simulink model "Sim_Multi"  (R2016b)
settings: Solver=ode3  StartTime=0.0  StopTime=sim_time  FixedStep=t_sim  MaxStep=t_control  RelTol=1e-5  EnableMultiTasking=on
values from neighbouring files (symbols this model uses):
  Att_init = [0;0;0] * d2r    [Init_Multi.m]
  Blade_flapping = 0    [Init_Multi.m]
  C_D = 0.40    (= 0.4)    [Init_Multi.m]
  CoG_nominal = [0;0;0.001]    [Init_Multi.m]
  CoG_real = [0;0;0.001]    [Init_Multi.m]
  Coriolis_correction = 1    [Init_Multi.m]
  d2r = pi/180    (= 0.0174532925199)    [Init_Multi.m]
  Dyn_thrust = 0    [Init_Multi.m]
  g = 9.80665    [Init_Multi.m]
  J_nominal = [Jxx Jxy Jxz;Jyx Jyy Jyz;Jzx Jzy Jzz]    [Init_Multi.m]
  J_real = [Jxx Jxy Jxz;Jyx Jyy Jyz;Jzx Jzy Jzz]    [Init_Multi.m]
  k1 = -1.125    [Init_Multi.m]
  k2 = -1.372    [Init_Multi.m]
  k3 = -1.718    [Init_Multi.m]
  k4 = -0.655    [Init_Multi.m]
  k_a1s = 1.5 / 4.0    (= 0.375)    [Init_Multi.m]
  k_beta = 0.23    [Init_Multi.m]
  kappa = 1.00    (= 1)    [Init_Multi.m]
  Kff_1 = 0.7*[1;1;0.95]    [Init_Multi.m]
  Ki_1 = 10*[1;1;1.5]    [Init_Multi.m]
  Kp_1 = 15*[1;1;1.5]    [Init_Multi.m]
  mass_nominal = 0.550    (= 0.55)    [Init_Multi.m]
  mass_real = 0.550    (= 0.55)    [Init_Multi.m]
  max_thrust = max_thrust + (MotorMatrix_nominal(i,7)*MotorMatrix_nominal(i,12)+MotorMatrix_nominal(i,8)*MotorMatrix_nominal(i,12)^2)    [Init_Multi.m]
  MaxRate_cmd = [360;360;120] * d2r    [Init_Multi.m]
  min_thrust = min_thrust + (MotorMatrix_nominal(i,7)*MotorMatrix_nominal(i,11)+MotorMatrix_nominal(i,8)*MotorMatrix_nominal(i,11)^2)    [Init_Multi.m]
  MotorMap = B' * inv(B * B')    [Init_Multi.m]
  MotorMatrix_nominal = [045 , 0.170 , -0.028 , -1 , 1.0 , 0.010 , [9.6820 , 0.010872]*1e-5 , [1.4504 , 0.0016312]*1e-6 , 0000 , 6000 , [0.0 , 0.0 , 0.0] , 8*2.54/100 , 11/1000;                         135 , 0.170 , -0.028 , +1 , 1.0 , 0.010 , [9.6820 , 0.010872]*1e-5 , [1.4504 , 0.0016312]*1e-6 , 0000 , 6000 , [0.0 , 0.0 , 0.0] , 8*2.54/100 , 11/1000;                         225 , 0.170 , -0.028 , -1 , 1.0 , 0.010 , [9. ...(+284 chars)    [Init_Multi.m]
  MotorMatrix_real = [045 , 0.170 , -0.028 , -1 , 1.0 , 0.010 , [9.6820 , 0.010872]*1e-5 , [1.4504 , 0.0016312]*1e-6 , 0000 , 6000 , [0.0 , 0.0 , 0.0] , 8*2.54/100 , 11/1000;                      135 , 0.170 , -0.028 , +1 , 1.0 , 0.010 , [9.6820 , 0.010872]*1e-5 , [1.4504 , 0.0016312]*1e-6 , 0000 , 6000 , [0.0 , 0.0 , 0.0] , 8*2.54/100 , 11/1000;                      225 , 0.170 , -0.028 , -1 , 1.0 , 0.010 , [9.6820 , ...(+275 chars)    [Init_Multi.m]
  Noise_flag = 0    [Init_Multi.m]
  omega_init = [0;0;0]    [Init_Multi.m]
  q_init = rpy2quat(Att_init)    [Init_Multi.m]
  r2d = 180/pi    (= 57.2957795131)    [Init_Multi.m]
  rho = 1.225    [Init_Multi.m]
  rpm2radpersec = 2*pi/60    (= 0.10471975512)    [Init_Multi.m]
  rpm_init = 3104.5025852    [Init_Multi.m]
  Surface_params = [a;b;c]    [Init_Multi.m]
  t_control = 1/500    (= 0.002)    [Init_Multi.m]
  t_sim = t_control/2    (= 0.001)    [Init_Multi.m]
  thrust_gain = (max_thrust - min_thrust) / 1000    (= 0)    [Init_Multi.m]
  thrust_offset = min_thrust    (= 0)    [Init_Multi.m]
  thrust_reserve = 0.10    (= 0.1)    [Init_Multi.m]
  v_h = 4.0    (= 4)    [Init_Multi.m]
  Vb_init = [0;0;0]    [Init_Multi.m]
  Vi_init = R_IB_init' * Vb_init    [Init_Multi.m]
  Xi_init = [0;0;0]    [Init_Multi.m]
undefined symbols (not defined in the file or in its folder): DiscIntNeverNeededParam, rpy2quat, thrust2rpm
libraries: simulink x17
(part 3 of 4)

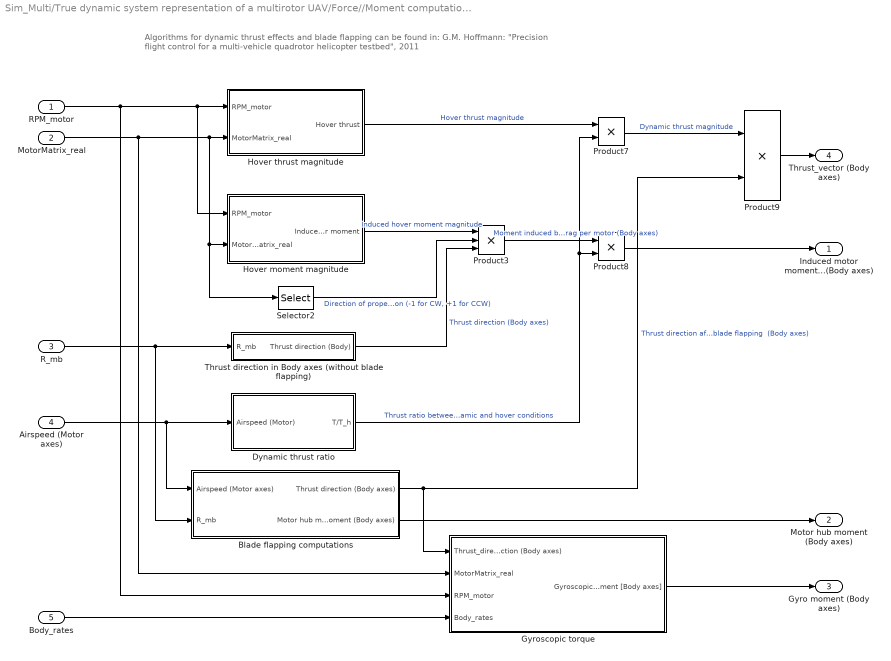
== system Sim_Multi/True dynamic system representation of a multirotor UAV/Force//Moment computation/Forces and moments generated by spinning propellers/For Each Subsystem/Thrust//moment vector for each propeller (Body axes)/Compute dynamic motor thrust and moments ==
  note: Algorithms for dynamic thrust effects and blade flapping can be found in:
      | G.M. Hoffmann: "Precision flight control for a multi-vehicle quadrotor helicopter testbed", 2011
  RPM_motor : Inport
  MotorMatrix_real : Inport  Port=2
  R_mb : Inport  Port=3
  Airspeed (Motor axes) : Inport  Port=4
  Body_rates : Inport  Port=5
  Blade flapping computations : Subsystem
  Dynamic thrust ratio : Subsystem
  Gyroscopic torque : Subsystem
  Hover moment magnitude : Subsystem
  Hover thrust magnitude : Subsystem
  Product3 : Product  Inputs=3
  Product7 : Product
  Product8 : Product
  Product9 : Product
  Selector2 : Selector  InputPortWidth=17  IndexOptions=Index vector (dialog)  Indices=[4]  OutputSizes=1
  Thrust direction in Body axes (without blade flapping) : Subsystem
  Induced motor moment (Body axes) : Outport
  Motor hub moment (Body axes) : Outport  Port=2
  Gyro moment (Body axes) : Outport  Port=3
  Thrust_vector (Body axes) : Outport  Port=4
  wires:
  RPM_motor/1 -> Gyroscopic torque/3(RPM_motor), Hover moment magnitude/1(RPM_motor), Hover thrust magnitude/1(RPM_motor)
  MotorMatrix_real/1 -> Gyroscopic torque/2(MotorMatrix_real), Selector2/1, Hover moment magnitude/2(MotorMatrix_real), Hover thrust magnitude/2(MotorMatrix_real)
  Selector2/1 -> Product3/2  "Direction of propeller rotation (-1 for CW, +1 for CCW)"
  Thrust direction in Body axes (without blade flapping)/1(Thrust direction (Body)) -> Product3/3  "Thrust direction (Body axes)"
  R_mb/1 -> Blade flapping computations/2(R_mb), Thrust direction in Body axes (without blade flapping)/1(R_mb)
  Airspeed (Motor axes)/1 -> Blade flapping computations/1(Airspeed (Motor axes)), Dynamic thrust ratio/1(Airspeed (Motor))
  Product3/1 -> Product8/1  "Moment induced by aerodynamic drag per motor (Body axes)"
  Product8/1 -> Induced motor moment (Body axes)/1
  Product7/1 -> Product9/1  "Dynamic thrust magnitude"
  Product9/1 -> Thrust_vector (Body axes)/1
  Blade flapping computations/1(Thrust direction (Body axes)) -> Gyroscopic torque/1(Thrust_direction (Body axes)), Product9/2  "Thrust direction after blade flapping  (Body axes)"
  Blade flapping computations/2(Motor hub moment (Body axes)) -> Motor hub moment (Body axes)/1
  Body_rates/1 -> Gyroscopic torque/4(Body_rates)
  Gyroscopic torque/1(Gyroscopic moment [Body axes]) -> Gyro moment (Body axes)/1
  Hover thrust magnitude/1(Hover thrust) -> Product7/1  "Hover thrust magnitude"
  Hover moment magnitude/1(Induced hover moment) -> Product3/1  "Induced hover moment magnitude"
  Dynamic thrust ratio/1(T/T_h) -> Product7/2, Product8/2  "Thrust ratio between dynamic and hover conditions"

== system Sim_Multi/True dynamic system representation of a multirotor UAV/Force//Moment computation/Forces and moments generated by spinning propellers/For Each Subsystem/Thrust//moment vector for each propeller (Body axes)/Coordinate transformation Body to Motor axes ==
  note: The true airspeed at prop computed here is the linear velocity (now in Motor axes)
      | with which this particular motor moves through the air.
      | So the point of view is: the surrounding air standing still and the airframe moving through it.
  MotorMatrix_real : Inport
  Airspeed (Body axes) : Inport  Port=2
  Conversion deg to rad : Gain  Gain=d2r
  Product : Product  Multiplication=Matrix(*)
  Rotation Matrix Body to Motor : Subsystem
  Selector : Selector  InputPortWidth=17  IndexOptions=Index vector (dialog)  Indices=[13 14 15]  OutputSizes=1
  R_mb : Outport
  Airspeed (Motor axes) : Outport  Port=2
  wires:
  Product/1 -> Airspeed (Motor axes)/1  "True airspeed at prop (Motor axes)"
  Rotation Matrix Body to Motor/1(R_mb) -> R_mb/1, Product/1  "Rotation matrix Body to Motor axes"
  MotorMatrix_real/1 -> Selector/1
  Selector/1 -> Conversion deg to rad/1
  Airspeed (Body axes)/1 -> Product/2  "True airspeed at prop (Body axes)"
  Conversion deg to rad/1 -> Rotation Matrix Body to Motor/1(Motor angles)

== system Sim_Multi/True dynamic system representation of a multirotor UAV/Force//Moment computation/Forces and moments generated by spinning propellers/For Each Subsystem/Thrust//moment vector for each propeller (Body axes)/Cross Product ==
  u : Inport
  v : Inport  Port=2
  Subsystem : Subsystem
  Subsystem1 : Subsystem
  Sum : Sum  Inputs=+|-
  u x v : Outport
  wires:
  Sum/1 -> u x v/1
  u/1 -> Subsystem1/1(u), Subsystem/1(u)
  v/1 -> Subsystem1/2(v), Subsystem/2(v)
  Subsystem/1(Positive elements) -> Sum/1
  Subsystem1/1(Negative elements) -> Sum/2

== system Sim_Multi/Controller/Controller Structure/Inner-loop control only/PI Rate controller/Gain Kff/Create diagonal 3x3 matrix/Subsystem9 ==
  C_11 : Inport  PortDimensions=1
  C_12 : Inport  Port=2  PortDimensions=1
  C_13 : Inport  Port=3  PortDimensions=1
  C_21 : Inport  Port=4  PortDimensions=1
  C_22 : Inport  Port=5  PortDimensions=1
  C_23 : Inport  Port=6  PortDimensions=1
  C_31 : Inport  Port=7  PortDimensions=1
  C_32 : Inport  Port=8  PortDimensions=1
  C_33 : Inport  Port=9  PortDimensions=1
  Reshape (9) to [3x3] column-major : Reshape  OutputDimensionality=Customize  OutputDimensions=[3,3]
  Vector Concatenate : Concatenate  NumInputs=9
  Diag : Outport
  wires:
  C_33/1 -> Vector Concatenate/9
  C_22/1 -> Vector Concatenate/5
  Reshape (9) to [3x3] column-major/1 -> Diag/1
  C_11/1 -> Vector Concatenate/1
  Vector Concatenate/1 -> Reshape (9) to [3x3] column-major/1
  C_32/1 -> Vector Concatenate/6
  C_31/1 -> Vector Concatenate/3
  C_21/1 -> Vector Concatenate/2
  C_13/1 -> Vector Concatenate/7
  C_12/1 -> Vector Concatenate/4
  C_23/1 -> Vector Concatenate/8

== system Sim_Multi/Controller/Controller Structure/Inner-loop control only/PI Rate controller/Gain Ki/Create diagonal 3x3 matrix/Subsystem9 ==
  C_11 : Inport  PortDimensions=1
  C_12 : Inport  Port=2  PortDimensions=1
  C_13 : Inport  Port=3  PortDimensions=1
  C_21 : Inport  Port=4  PortDimensions=1
  C_22 : Inport  Port=5  PortDimensions=1
  C_23 : Inport  Port=6  PortDimensions=1
  C_31 : Inport  Port=7  PortDimensions=1
  C_32 : Inport  Port=8  PortDimensions=1
  C_33 : Inport  Port=9  PortDimensions=1
  Reshape (9) to [3x3] column-major : Reshape  OutputDimensionality=Customize  OutputDimensions=[3,3]
  Vector Concatenate : Concatenate  NumInputs=9
  Diag : Outport
  wires:
  C_33/1 -> Vector Concatenate/9
  C_22/1 -> Vector Concatenate/5
  Reshape (9) to [3x3] column-major/1 -> Diag/1
  C_11/1 -> Vector Concatenate/1
  Vector Concatenate/1 -> Reshape (9) to [3x3] column-major/1
  C_32/1 -> Vector Concatenate/6
  C_31/1 -> Vector Concatenate/3
  C_21/1 -> Vector Concatenate/2
  C_13/1 -> Vector Concatenate/7
  C_12/1 -> Vector Concatenate/4
  C_23/1 -> Vector Concatenate/8

== system Sim_Multi/Controller/Controller Structure/Inner-loop control only/PI Rate controller/Gain Kp/Create diagonal 3x3 matrix/Subsystem9 ==
  C_11 : Inport  PortDimensions=1
  C_12 : Inport  Port=2  PortDimensions=1
  C_13 : Inport  Port=3  PortDimensions=1
  C_21 : Inport  Port=4  PortDimensions=1
  C_22 : Inport  Port=5  PortDimensions=1
  C_23 : Inport  Port=6  PortDimensions=1
  C_31 : Inport  Port=7  PortDimensions=1
  C_32 : Inport  Port=8  PortDimensions=1
  C_33 : Inport  Port=9  PortDimensions=1
  Reshape (9) to [3x3] column-major : Reshape  OutputDimensionality=Customize  OutputDimensions=[3,3]
  Vector Concatenate : Concatenate  NumInputs=9
  Diag : Outport
  wires:
  C_33/1 -> Vector Concatenate/9
  C_22/1 -> Vector Concatenate/5
  Reshape (9) to [3x3] column-major/1 -> Diag/1
  C_11/1 -> Vector Concatenate/1
  Vector Concatenate/1 -> Reshape (9) to [3x3] column-major/1
  C_32/1 -> Vector Concatenate/6
  C_31/1 -> Vector Concatenate/3
  C_21/1 -> Vector Concatenate/2
  C_13/1 -> Vector Concatenate/7
  C_12/1 -> Vector Concatenate/4
  C_23/1 -> Vector Concatenate/8

== system Sim_Multi/True dynamic system representation of a multirotor UAV/Force//Moment computation/Compute aerodynamic drag of the airframe in Body axes/Aerodynamic drag force/Nonzero airspeed/Normalize/norm ==
  u : Inport
  Complex to Real-Imag : ComplexToRealImag  Output=Real
  Sqrt : Sqrt  SaturateOnIntegerOverflow=on
  dot_product : Subsystem
  ||u|| : Outport
  wires:
  u/1 -> dot_product/1(u), dot_product/2(v)
  dot_product/1(u.v) -> Sqrt/1
  Sqrt/1 -> Complex to Real-Imag/1
  Complex to Real-Imag/1 -> ||u||/1

== system Sim_Multi/True dynamic system representation of a multirotor UAV/Force//Moment computation/Compute aerodynamic drag of the airframe in Body axes/Aerodynamic drag force/Nonzero airspeed/Surface area computation/Scaling factor computation ==
  Airspeed (Body) : Inport
  Surface_params : Inport  Port=2
  Add : Sum  Inputs=+++
  Demux : Demux  Outputs=3
  Demux1 : Demux  Outputs=3
  Divide : Product  Inputs=*/
  Divide1 : Product  Inputs=*/
  Divide2 : Product  Inputs=*/
  Product : Product
  Product1 : Product
  Product2 : Product
  Reciprocal Sqrt : Sqrt  Operator=rSqrt  SaturateOnIntegerOverflow=on
  Scaling factor : Outport
  wires:
  Divide2/1 -> Product2/2, Product2/1
  Reciprocal Sqrt/1 -> Scaling factor/1
  Demux1/3 -> Divide2/2  "c"
  Demux/3 -> Divide2/1  "z"
  Divide/1 -> Product/2, Product/1
  Airspeed (Body)/1 -> Demux/1
  Surface_params/1 -> Demux1/1
  Demux1/1 -> Divide/2  "a"
  Demux/1 -> Divide/1  "x"
  Product/1 -> Add/1
  Product2/1 -> Add/3
  Add/1 -> Reciprocal Sqrt/1
  Demux/2 -> Divide1/1  "y"
  Divide1/1 -> Product1/2, Product1/1
  Demux1/2 -> Divide1/2  "b"
  Product1/1 -> Add/2

== system Sim_Multi/True dynamic system representation of a multirotor UAV/Force//Moment computation/Compute aerodynamic drag of the airframe in Body axes/Aerodynamic drag force/Nonzero airspeed/Surface area computation/Surface area computation ==
  Airspeed (Body) : Inport
  Scaling factor : Inport  Port=2
  Product : Product
  norm : Subsystem
  Surface area : Outport
  wires:
  Scaling factor/1 -> Product/2
  Airspeed (Body)/1 -> Product/1
  Product/1 -> norm/1(u)
  norm/1(||u||) -> Surface area/1

== system Sim_Multi/True dynamic system representation of a multirotor UAV/Force//Moment computation/Compute aerodynamic drag of the airframe in Body axes/Aerodynamic drag force/Nonzero airspeed/u^2/dot_product ==
  u : Inport
  v : Inport  Port=2
  Product : Product  Multiplication=Matrix(*)  RndMeth=Zero
  Reshape : Reshape  OutputDimensionality=Column vector (2-D)
  Reshape1 : Reshape  OutputDimensionality=Column vector (2-D)
  transpose : Math  Operator=transpose  SaturateOnIntegerOverflow=on
  u.v : Outport
  wires:
  v/1 -> Reshape1/1
  u/1 -> Reshape/1
  Reshape/1 -> transpose/1
  transpose/1 -> Product/1
  Reshape1/1 -> Product/2
  Product/1 -> u.v/1

== system Sim_Multi/True dynamic system representation of a multirotor UAV/Force//Moment computation/Forces and moments generated by spinning propellers/For Each Subsystem/Thrust//moment vector for each propeller (Body axes)/Compute dynamic motor thrust and moments/Blade flapping computations ==
  note: Blade flapping computations are motivated by algorithms found in:
      | G.M. Hoffmann: "Precision flight control for a multi-vehicle quadrotor helicopter testbed", 2011
      | The idea is the following:
      | The thrust vector is tilted backwards from the direction of motion. The amount of tilt depends on the magnitude of the airspeed vector in the (untilted) propeller plane.
      | The tilt direction is in the plane defined by the airspeed xy vector and the (untilted) thrust vector in Motor axes.
      | The normal vector to this plane can be found by computing the cross product of untilted thrust vector and airspeed xy vector.
      | The new (tilted) thrust vector can then be found by applying the Rodrigues rotation formula, see Wikipedia
  Airspeed (Motor axes) : Inport
  R_mb : Inport  Port=2
  Demux4 : Demux  Outputs=[2,1]
  If : If  IfExpression=u1 == 0
  Merge : Merge
  Merge1 : Merge
  Nonzero airspeed in rotor plane : Subsystem  TreatAsAtomicUnit=on
  Terminator : Terminator
  Zero airspeed in rotor plane : Subsystem  TreatAsAtomicUnit=on
  norm : Subsystem
  Thrust direction (Body axes) : Outport
  Motor hub moment (Body axes) : Outport  Port=2
  wires:
  If/1 -> Zero airspeed in rotor plane/Action
  Zero airspeed in rotor plane/1(Thrust direction (Body)) -> Merge/1
  Nonzero airspeed in rotor plane/1(Thrust direction (Body)) -> Merge/2
  If/2 -> Nonzero airspeed in rotor plane/Action
  Airspeed (Motor axes)/1 -> Demux4/1
  Demux4/2 -> Terminator/1  "Airspeed component along motor shaft"
  Demux4/1 -> norm/1(u), Zero airspeed in rotor plane/1(Airspeed xy), Nonzero airspeed in rotor plane/1(Airspeed xy)  "Airspeed components in (unbent) rotor plane"
  norm/1(||u||) -> If/1  "Airspeed xy component  magnitude"
  Merge/1 -> Thrust direction (Body axes)/1  "New tilted thrust direction (Body axes) (This is a unit vector)"
  R_mb/1 -> Nonzero airspeed in rotor plane/2(R_mb), Zero airspeed in rotor plane/2(R_mb)
  Merge1/1 -> Motor hub moment (Body axes)/1  "Moment in the motor hub due to bending of the propeller (Body axes)"
  Zero airspeed in rotor plane/2(Hub moment (Body)) -> Merge1/1
  Nonzero airspeed in rotor plane/2(Hub moment (Body)) -> Merge1/2

== system Sim_Multi/True dynamic system representation of a multirotor UAV/Force//Moment computation/Forces and moments generated by spinning propellers/For Each Subsystem/Thrust//moment vector for each propeller (Body axes)/Compute dynamic motor thrust and moments/Dynamic thrust ratio ==
  Airspeed (Motor) : Inport
  Angle of attack and airspeed magnitude : Subsystem
  Compute the climb speed : Subsystem
  Constant : Constant
  Constant1 : Constant  Value=Dyn_thrust
  Divide : Product  Inputs=*/
  Flight modes of the propeller : Subsystem
  Induced velocity at hover : Constant  Value=v_h
  Product2 : Product
  Sum2 : Sum  Inputs=|+-
  Switch : Switch  Criteria=u2 > Threshold  Threshold=0.5
  Trigonometric Function : Trigonometry
  T/T_h : Outport
  wires:
  Airspeed (Motor)/1 -> Angle of attack and airspeed magnitude/1(Airspeed (Motor axes)), Compute the climb speed/1(Airspeed (Motor axes))
  Trigonometric Function/1 -> Product2/1
  Sum2/1 -> Divide/2
  Angle of attack and airspeed magnitude/2(Airspeed magnitude) -> Product2/2  "Airspeed magnitude v_inf"
  Angle of attack and airspeed magnitude/1(AoA (rad)) -> Trigonometric Function/1  "Angle of Attack"
  Compute the climb speed/1(v_c) -> Flight modes of the propeller/2(v_c)
  Flight modes of the propeller/1(v_i) -> Sum2/1
  Product2/1 -> Sum2/2
  Induced velocity at hover/1 -> Divide/1, Flight modes of the propeller/1(v_h)
  Switch/1 -> T/T_h/1  "Thrust ratio T/T_h"
  Divide/1 -> Switch/1
  Constant/1 -> Switch/3
  Constant1/1 -> Switch/2

== system Sim_Multi/True dynamic system representation of a multirotor UAV/Force//Moment computation/Forces and moments generated by spinning propellers/For Each Subsystem/Thrust//moment vector for each propeller (Body axes)/Compute dynamic motor thrust and moments/Gyroscopic torque ==
  note: The thrust direction chosen here is the one after the effects of blade flapping.
      | The reasoning being that the propeller is bent in that direction and therefore
      | a majority of its moment of inertia effects will act in that direction as well (even
      | though the motor is not affected by blade flapping).
  Thrust_direction (Body axes) : Inport
  MotorMatrix_real : Inport  Port=2
  RPM_motor : Inport  Port=3
  Body_rates : Inport  Port=4
  Conversion rpm to rad/s : Gain  Gain=rpm2radpersec
  Cross Product : Subsystem
  Product5 : Product  Inputs=4
  Propeller moment of inertia : Subsystem
  Reshape1 : Reshape  OutputDimensionality=Column vector (2-D)
  Reshape2 : Reshape  OutputDimensionality=Row vector (2-D)
  Selector6 : Selector  InputPortWidth=17  IndexOptions=Index vector (dialog)  Indices=[4]  OutputSizes=1
  Gyroscopic moment [Body axes] : Outport
  wires:
  Body_rates/1 -> Reshape2/1
  Product5/1 -> Reshape1/1
  Cross Product/1(u x v) -> Product5/3
  Propeller moment of inertia/1(Out1) -> Product5/1  "Moment of inertia for each propeller"
  Selector6/1 -> Product5/2  "Direction of propeller rotation (+1 for CW, -1 for CCW)"
  Conversion rpm to rad/s/1 -> Product5/4
  RPM_motor/1 -> Conversion rpm to rad/s/1
  MotorMatrix_real/1 -> Selector6/1, Propeller moment of inertia/1(In1)
  Thrust_direction (Body axes)/1 -> Cross Product/2(v)  "Thrust direction (Body axes)"
  Reshape2/1 -> Cross Product/1(u)
  Reshape1/1 -> Gyroscopic moment [Body axes]/1

== system Sim_Multi/True dynamic system representation of a multirotor UAV/Force//Moment computation/Forces and moments generated by spinning propellers/For Each Subsystem/Thrust//moment vector for each propeller (Body axes)/Compute dynamic motor thrust and moments/Hover moment magnitude ==
  RPM_motor : Inport
  MotorMatrix_real : Inport  Port=2
  Product : Product
  Product1 : Product  Inputs=3
  Selector : Selector  InputPortWidth=17  IndexOptions=Index vector (dialog)  Indices=[9]  OutputSizes=1
  Selector1 : Selector  InputPortWidth=17  IndexOptions=Index vector (dialog)  Indices=[10]  OutputSizes=1
  Sum : Sum  Inputs=|++
  Induced hover moment : Outport
  wires:
  Selector/1 -> Product/2  "Linear torque parameter b1"
  Selector1/1 -> Product1/3  "Quadratic torque parameter b2"
  Product1/1 -> Sum/2
  Product/1 -> Sum/1
  Sum/1 -> Induced hover moment/1  "Motor torque magnitude"
  RPM_motor/1 -> Product/1, Product1/1, Product1/2
  MotorMatrix_real/1 -> Selector1/1, Selector/1

== system Sim_Multi/True dynamic system representation of a multirotor UAV/Force//Moment computation/Forces and moments generated by spinning propellers/For Each Subsystem/Thrust//moment vector for each propeller (Body axes)/Compute dynamic motor thrust and moments/Hover thrust magnitude ==
  RPM_motor : Inport
  MotorMatrix_real : Inport  Port=2
  Product4 : Product
  Product5 : Product
  Product6 : Product
  Selector3 : Selector  InputPortWidth=17  IndexOptions=Index vector (dialog)  Indices=[7]  OutputSizes=1
  Selector4 : Selector  InputPortWidth=17  IndexOptions=Index vector (dialog)  Indices=[8]  OutputSizes=1
  Sum1 : Sum  Inputs=|++
  Hover thrust : Outport
  wires:
  Selector4/1 -> Product6/2  "Quadratic thrust parameter a2"
  Selector3/1 -> Product4/2  "Linear thrust parameter a1"
  Product6/1 -> Sum1/2
  Product5/1 -> Product6/1
  Product4/1 -> Sum1/1
  Sum1/1 -> Hover thrust/1  "Hover thrust magnitude"
  MotorMatrix_real/1 -> Selector4/1, Selector3/1
  RPM_motor/1 -> Product4/1, Product5/1, Product5/2

== system Sim_Multi/True dynamic system representation of a multirotor UAV/Force//Moment computation/Forces and moments generated by spinning propellers/For Each Subsystem/Thrust//moment vector for each propeller (Body axes)/Compute dynamic motor thrust and moments/Thrust direction in Body axes (without blade flapping) ==
  R_mb : Inport
  Constant : Constant  Value=[0;0;-1]
  Math Function : Math  Operator=transpose  SaturateOnIntegerOverflow=on
  Product9 : Product  Multiplication=Matrix(*)
  Reshape5 : Reshape  OutputDimensionality=Column vector (2-D)
  Thrust direction (Body) : Outport
  wires:
  Reshape5/1 -> Thrust direction (Body)/1
  Product9/1 -> Reshape5/1
  R_mb/1 -> Math Function/1  "Rotation matrix Body to Motor axes"
  Constant/1 -> Product9/2  "Thrust direction vector (Motor axes)"
  Math Function/1 -> Product9/1

== system Sim_Multi/True dynamic system representation of a multirotor UAV/Force//Moment computation/Forces and moments generated by spinning propellers/For Each Subsystem/Thrust//moment vector for each propeller (Body axes)/Coordinate transformation Body to Motor axes/Rotation Matrix Body to Motor ==
  note: This is the rotation matrix R_123 as described in:
      | J. Diebel: "Representing Attitude: Euler Angles, Unit Quaternions, and Rotation Vectors", 10/20/2006
  Motor angles : Inport
  Subsystem : Subsystem
  Subsystem1 : Subsystem
  Subsystem2 : Subsystem
  Subsystem3 : Subsystem
  Subsystem4 : Subsystem
  Subsystem5 : Subsystem
  Subsystem6 : Subsystem
  Subsystem7 : Subsystem
  Subsystem8 : Subsystem
  Subsystem9 : Subsystem
  R_mb : Outport
  wires:
  Motor angles/1 -> Subsystem1/1(Euler), Subsystem2/1(Euler), Subsystem3/1(Euler), Subsystem4/1(Euler), Subsystem5/1(Euler), Subsystem6/1(Euler), Subsystem8/1(Euler), Subsystem7/1(Euler), Subsystem/1(Euler)
  Subsystem/1(R_11) -> Subsystem9/1(R_11)
  Subsystem1/1(R_12) -> Subsystem9/2(R_12)
  Subsystem2/1(R_13) -> Subsystem9/3(R_13)
  Subsystem3/1(R_21) -> Subsystem9/4(R_21)
  Subsystem4/1(R_22) -> Subsystem9/5(R_22)
  Subsystem8/1(R_33) -> Subsystem9/9(R_33)
  Subsystem7/1(R_32) -> Subsystem9/8(R_32)
  Subsystem6/1(R_31) -> Subsystem9/7(R_31)
  Subsystem5/1(R_23) -> Subsystem9/6(R_23)
  Subsystem9/1(R_mb) -> R_mb/1

== system Sim_Multi/True dynamic system representation of a multirotor UAV/Force//Moment computation/Forces and moments generated by spinning propellers/For Each Subsystem/Thrust//moment vector for each propeller (Body axes)/Cross Product/Subsystem ==
  u : Inport
  v : Inport  Port=2
  Demux : Demux  Outputs=3
  Demux1 : Demux  Outputs=3
  Mux : Mux  Inputs=3
  Product : Product
  Product1 : Product
  Product2 : Product
  Positive elements : Outport
  wires:
  Mux/1 -> Positive elements/1
  v/1 -> Demux1/1
  u/1 -> Demux/1
  Demux/2 -> Product/1
  Demux1/3 -> Product/2
  Demux/3 -> Product1/1
  Demux1/1 -> Product1/2
  Demux/1 -> Product2/1
  Demux1/2 -> Product2/2
  Product/1 -> Mux/1
  Product1/1 -> Mux/2
  Product2/1 -> Mux/3

== system Sim_Multi/True dynamic system representation of a multirotor UAV/Force//Moment computation/Forces and moments generated by spinning propellers/For Each Subsystem/Thrust//moment vector for each propeller (Body axes)/Cross Product/Subsystem1 ==
  u : Inport
  v : Inport  Port=2
  Demux : Demux  Outputs=3
  Demux1 : Demux  Outputs=3
  Mux : Mux  Inputs=3
  Product : Product
  Product1 : Product
  Product2 : Product
  Negative elements : Outport
  wires:
  Mux/1 -> Negative elements/1
  v/1 -> Demux1/1
  u/1 -> Demux/1
  Product/1 -> Mux/1
  Product1/1 -> Mux/2
  Product2/1 -> Mux/3
  Demux/3 -> Product/1
  Demux1/2 -> Product/2
  Demux/1 -> Product1/1
  Demux1/3 -> Product1/2
  Demux/2 -> Product2/1
  Demux1/1 -> Product2/2

== system Sim_Multi/True dynamic system representation of a multirotor UAV/Force//Moment computation/Compute aerodynamic drag of the airframe in Body axes/Aerodynamic drag force/Nonzero airspeed/Normalize/norm/dot_product ==
  u : Inport
  v : Inport  Port=2
  Product : Product  Multiplication=Matrix(*)  RndMeth=Zero
  Reshape : Reshape  OutputDimensionality=Column vector (2-D)
  Reshape1 : Reshape  OutputDimensionality=Column vector (2-D)
  transpose : Math  Operator=transpose  SaturateOnIntegerOverflow=on
  u.v : Outport
  wires:
  v/1 -> Reshape1/1
  u/1 -> Reshape/1
  Reshape/1 -> transpose/1
  transpose/1 -> Product/1
  Reshape1/1 -> Product/2
  Product/1 -> u.v/1

== system Sim_Multi/True dynamic system representation of a multirotor UAV/Force//Moment computation/Compute aerodynamic drag of the airframe in Body axes/Aerodynamic drag force/Nonzero airspeed/Surface area computation/Surface area computation/norm ==
  u : Inport
  Complex to Real-Imag : ComplexToRealImag  Output=Real
  Sqrt : Sqrt  SaturateOnIntegerOverflow=on
  dot_product : Subsystem
  ||u|| : Outport
  wires:
  u/1 -> dot_product/1(u), dot_product/2(v)
  dot_product/1(u.v) -> Sqrt/1
  Sqrt/1 -> Complex to Real-Imag/1
  Complex to Real-Imag/1 -> ||u||/1

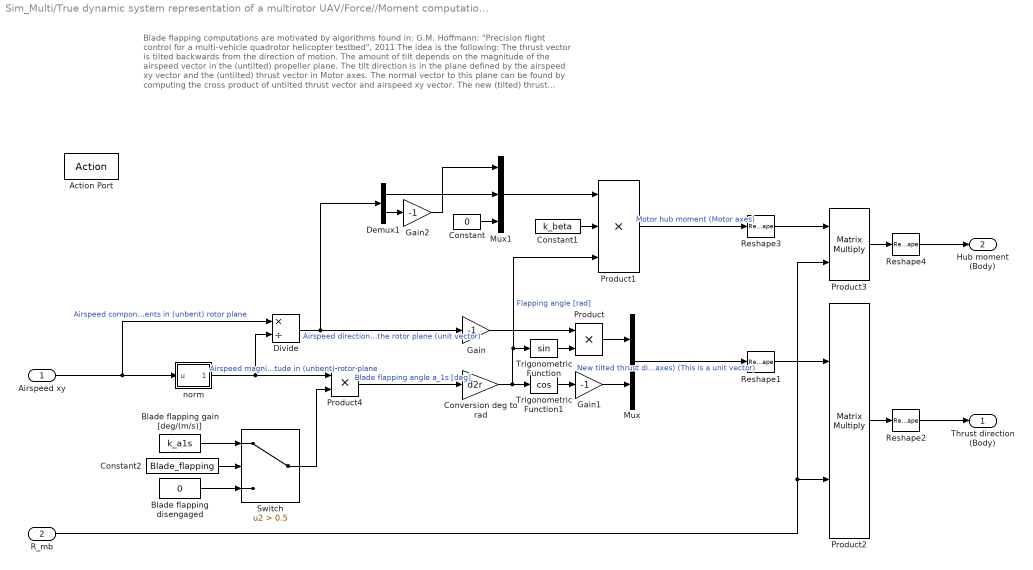
== system Sim_Multi/True dynamic system representation of a multirotor UAV/Force//Moment computation/Forces and moments generated by spinning propellers/For Each Subsystem/Thrust//moment vector for each propeller (Body axes)/Compute dynamic motor thrust and moments/Blade flapping computations/Nonzero airspeed in rotor plane ==
  note: Blade flapping computations are motivated by algorithms found in:
      | G.M. Hoffmann: "Precision flight control for a multi-vehicle quadrotor helicopter testbed", 2011
      | The idea is the following:
      | The thrust vector is tilted backwards from the direction of motion. The amount of tilt depends on the magnitude of the airspeed vector in the (untilted) propeller plane.
      | The tilt direction is in the plane defined by the airspeed xy vector and the (untilted) thrust vector in Motor axes.
      | The normal vector to this plane can be found by computing the cross product of untilted thrust vector and airspeed xy vector.
      | The new (tilted) thrust vector can then be found by applying the Rodrigues rotation formula, see Wikipedia
  Airspeed xy : Inport
  R_mb : Inport  Port=2
  Action Port : ActionPort  ActionType=else
  Blade flapping disengaged : Constant  Value=0
  Blade flapping gain [deg/(m/s)] : Constant  Value=k_a1s
  Constant : Constant  Value=0
  Constant1 : Constant  Value=k_beta
  Constant2 : Constant  Value=Blade_flapping
  Conversion deg to rad : Gain  Gain=d2r
  Demux1 : Demux  Outputs=2
  Divide : Product  Inputs=*/
  Gain : Gain  Gain=-1
  Gain1 : Gain  Gain=-1
  Gain2 : Gain  Gain=-1
  Mux : Mux  Inputs=2
  Mux1 : Mux  Inputs=3
  Product : Product
  Product1 : Product  Inputs=3
  Product2 : Product  Multiplication=Matrix(*)
  Product3 : Product  Multiplication=Matrix(*)
  Product4 : Product
  Reshape1 : Reshape  OutputDimensionality=Row vector (2-D)
  Reshape2 : Reshape  OutputDimensionality=Column vector (2-D)
  Reshape3 : Reshape  OutputDimensionality=Row vector (2-D)
  Reshape4 : Reshape  OutputDimensionality=Column vector (2-D)
  Switch : Switch  Criteria=u2 > Threshold  Threshold=0.5
  Trigonometric Function : Trigonometry
  Trigonometric Function1 : Trigonometry  Operator=cos
  norm : Subsystem
  Thrust direction (Body) : Outport
  Hub moment (Body) : Outport  Port=2
  wires:
  Airspeed xy/1 -> Divide/1, norm/1(u)  "Airspeed components in (unbent) rotor plane"
  norm/1(||u||) -> Product4/1, Divide/2  "Airspeed magnitude in (unbent) rotor plane"
  Product4/1 -> Conversion deg to rad/1  "Blade flapping angle a_1s [deg]"
  Trigonometric Function/1 -> Product/2
  Product/1 -> Mux/1
  Trigonometric Function1/1 -> Gain1/1
  Gain1/1 -> Mux/2
  Conversion deg to rad/1 -> Product1/3, Trigonometric Function/1, Trigonometric Function1/1  "Flapping angle [rad]"
  Mux/1 -> Reshape1/1  "New tilted thrust direction vector (Motor axes) (This is a unit vector)"
  Divide/1 -> Demux1/1, Gain/1  "Airspeed direction in the rotor plane (unit vector)"
  Gain/1 -> Product/1
  Product2/1 -> Reshape2/1
  Reshape2/1 -> Thrust direction (Body)/1
  Reshape1/1 -> Product2/1
  R_mb/1 -> Product2/2, Product3/2
  Constant1/1 -> Product1/2
  Demux1/2 -> Gain2/1
  Gain2/1 -> Mux1/1
  Demux1/1 -> Mux1/2
  Constant/1 -> Mux1/3
  Mux1/1 -> Product1/1
  Product1/1 -> Reshape3/1  "Motor hub moment (Motor axes)"
  Product3/1 -> Reshape4/1
  Reshape4/1 -> Hub moment (Body)/1
  Reshape3/1 -> Product3/1
  Constant2/1 -> Switch/2
  Blade flapping gain [deg/(m/s)]/1 -> Switch/1
  Blade flapping disengaged/1 -> Switch/3
  Switch/1 -> Product4/2

== system Sim_Multi/True dynamic system representation of a multirotor UAV/Force//Moment computation/Forces and moments generated by spinning propellers/For Each Subsystem/Thrust//moment vector for each propeller (Body axes)/Compute dynamic motor thrust and moments/Blade flapping computations/Zero airspeed in rotor plane ==
  Airspeed xy : Inport
  R_mb : Inport  Port=2
  Action Port : ActionPort  ActionType=then
  Constant : Constant  Value=[0;0;-1]
  Constant1 : Constant  Value=[0;0;0]
  Terminator : Terminator
  Terminator1 : Terminator
  Thrust direction (Body) : Outport  InitialOutput=[0;0;-1]
  Hub moment (Body) : Outport  Port=2  InitialOutput=[0;0;0]
  wires:
  Airspeed xy/1 -> Terminator/1  "Airspeed components in (unbent) rotor plane"
  Constant/1 -> Thrust direction (Body)/1
  Constant1/1 -> Hub moment (Body)/1
  R_mb/1 -> Terminator1/1

== system Sim_Multi/True dynamic system representation of a multirotor UAV/Force//Moment computation/Forces and moments generated by spinning propellers/For Each Subsystem/Thrust//moment vector for each propeller (Body axes)/Compute dynamic motor thrust and moments/Blade flapping computations/norm ==
  u : Inport
  Complex to Real-Imag : ComplexToRealImag  Output=Real
  Sqrt : Sqrt  SaturateOnIntegerOverflow=on
  dot_product : Subsystem
  ||u|| : Outport
  wires:
  u/1 -> dot_product/1(u), dot_product/2(v)
  dot_product/1(u.v) -> Sqrt/1
  Sqrt/1 -> Complex to Real-Imag/1
  Complex to Real-Imag/1 -> ||u||/1

== system Sim_Multi/True dynamic system representation of a multirotor UAV/Force//Moment computation/Forces and moments generated by spinning propellers/For Each Subsystem/Thrust//moment vector for each propeller (Body axes)/Compute dynamic motor thrust and moments/Dynamic thrust ratio/Angle of attack and airspeed magnitude ==
  note: In this context, Angle of Attack is defined as zero when the airspeed lies in the propeller plane.
      | Angle of Attack increases positively when pitching up.
      | Thus, flying straight up in windless conditions would equal an AoA of -90 degrees.
      | Descending straight down in windless conditions would equal an AoA of +90 degrees.
  Airspeed (Motor axes) : Inport
  If : If  IfExpression=u1 == 0
  Merge : Merge
  Nonzero airspeed : Subsystem  TreatAsAtomicUnit=on
  Zero airspeed : Subsystem  TreatAsAtomicUnit=on
  norm2 : Subsystem
  AoA (rad) : Outport
  Airspeed magnitude : Outport  Port=2
  wires:
  If/1 -> Zero airspeed/Action
  Zero airspeed/1(AoA (rad)) -> Merge/1
  Nonzero airspeed/1(AoA (rad)) -> Merge/2
  If/2 -> Nonzero airspeed/Action
  Airspeed (Motor axes)/1 -> norm2/1(u), Nonzero airspeed/1(Airspeed (Motor)), Zero airspeed/1(Airspeed (Motor))
  Merge/1 -> AoA (rad)/1  "Angle of attack (rad)"
  norm2/1(||u||) -> Airspeed magnitude/1, If/1  "Airspeed magnitude"

== system Sim_Multi/True dynamic system representation of a multirotor UAV/Force//Moment computation/Forces and moments generated by spinning propellers/For Each Subsystem/Thrust//moment vector for each propeller (Body axes)/Compute dynamic motor thrust and moments/Dynamic thrust ratio/Compute the climb speed ==
  note: This block determines the climb speed v_c
      | Since the motor coordinate system has its z-axis (along the motor axis) pointing down,
      | a positive z-velocity would mean sinking. Therefore the negative sign.
  Airspeed (Motor axes) : Inport
  Demux : Demux  Outputs=3
  Gain : Gain  Gain=-1
  Terminator : Terminator
  Terminator1 : Terminator
  v_c : Outport
  wires:
  Gain/1 -> v_c/1  "Climb speed v_c"
  Demux/1 -> Terminator/1
  Airspeed (Motor axes)/1 -> Demux/1
  Demux/2 -> Terminator1/1
  Demux/3 -> Gain/1

== system Sim_Multi/True dynamic system representation of a multirotor UAV/Force//Moment computation/Forces and moments generated by spinning propellers/For Each Subsystem/Thrust//moment vector for each propeller (Body axes)/Compute dynamic motor thrust and moments/Dynamic thrust ratio/Flight modes of the propeller ==
  v_h : Inport
  v_c : Inport  Port=2
  Divide : Product  Inputs=*/  SampleTime=t_sim
  If : If  IfExpression=u1 >= 0  ElseIfExpressions=u1 >= -2  SampleTime=t_sim
  Merge : Merge  Inputs=3
  Normal working state vc/vh >= 0 : Subsystem  TreatAsAtomicUnit=on
  "Vortex ring state -2 <= vc/vh < 0 " : Subsystem  TreatAsAtomicUnit=on
  Windmill braking state vc/vh < -2 : Subsystem  TreatAsAtomicUnit=on
  v_i : Outport
  wires:
  Merge/1 -> v_i/1
  v_c/1 -> Windmill braking state vc/vh < -2/1(v_c), "Vortex ring state -2 <= vc/vh < 0 "/1(v_c), Normal working state vc/vh >= 0/1(v_c), Divide/1
  v_h/1 -> Divide/2
  Divide/1 -> If/1  "v_c/v_h"
  If/1 -> Normal working state vc/vh >= 0/Action
  Normal working state vc/vh >= 0/1(v_i) -> Merge/1
  "Vortex ring state -2 <= vc/vh < 0 "/1(v_i) -> Merge/2
  Windmill braking state vc/vh < -2/1(v_i) -> Merge/3
  If/2 -> "Vortex ring state -2 <= vc/vh < 0 "/Action
  If/3 -> Windmill braking state vc/vh < -2/Action

== system Sim_Multi/True dynamic system representation of a multirotor UAV/Force//Moment computation/Forces and moments generated by spinning propellers/For Each Subsystem/Thrust//moment vector for each propeller (Body axes)/Compute dynamic motor thrust and moments/Gyroscopic torque/Cross Product ==
  u : Inport
  v : Inport  Port=2
  Subsystem : Subsystem
  Subsystem1 : Subsystem
  Sum : Sum  Inputs=+|-
  u x v : Outport
  wires:
  Sum/1 -> u x v/1
  u/1 -> Subsystem1/1(u), Subsystem/1(u)
  v/1 -> Subsystem1/2(v), Subsystem/2(v)
  Subsystem/1(Positive elements) -> Sum/1
  Subsystem1/1(Negative elements) -> Sum/2

== system Sim_Multi/True dynamic system representation of a multirotor UAV/Force//Moment computation/Forces and moments generated by spinning propellers/For Each Subsystem/Thrust//moment vector for each propeller (Body axes)/Compute dynamic motor thrust and moments/Gyroscopic torque/Propeller moment of inertia ==
  note: This computes the approximate moment of inertia of a propeller given its mass and diameter.
      | It is the mean value of the disk approximation and the rod approximation for a spinning propeller.
  In1 : Inport
  Gain : Gain  Gain=0.5
  Gain1 : Gain  Gain=7/12
  Product7 : Product  Inputs=3
  Selector4 : Selector  InputPortWidth=17  IndexOptions=Index vector (dialog)  Indices=[16]  OutputSizes=1
  Selector5 : Selector  InputPortWidth=17  IndexOptions=Index vector (dialog)  Indices=[17]  OutputSizes=1
  Out1 : Outport
  wires:
  Selector5/1 -> Product7/3  "Propeller mass"
  Gain/1 -> Product7/2, Product7/1
  In1/1 -> Selector5/1, Selector4/1
  Selector4/1 -> Gain/1  "Propeller diameter"
  Gain1/1 -> Out1/1
  Product7/1 -> Gain1/1

== system Sim_Multi/True dynamic system representation of a multirotor UAV/Force//Moment computation/Forces and moments generated by spinning propellers/For Each Subsystem/Thrust//moment vector for each propeller (Body axes)/Coordinate transformation Body to Motor axes/Rotation Matrix Body to Motor/Subsystem ==
  Euler : Inport
  Demux : Demux  Outputs=3
  Product : Product
  Terminator : Terminator
  Trigonometric Function1 : Trigonometry  Operator=cos
  Trigonometric Function3 : Trigonometry  Operator=cos
  R_11 : Outport
  wires:
  Euler/1 -> Demux/1
  Demux/1 -> Terminator/1  "phi"
  Demux/2 -> Trigonometric Function1/1  "theta"
  Demux/3 -> Trigonometric Function3/1  "psi"
  Trigonometric Function1/1 -> Product/1
  Trigonometric Function3/1 -> Product/2
  Product/1 -> R_11/1

== system Sim_Multi/True dynamic system representation of a multirotor UAV/Force//Moment computation/Forces and moments generated by spinning propellers/For Each Subsystem/Thrust//moment vector for each propeller (Body axes)/Coordinate transformation Body to Motor axes/Rotation Matrix Body to Motor/Subsystem1 ==
  Euler : Inport
  Demux : Demux  Outputs=3
  Product : Product
  Terminator : Terminator
  Trigonometric Function1 : Trigonometry  Operator=cos
  Trigonometric Function3 : Trigonometry
  R_12 : Outport
  wires:
  Euler/1 -> Demux/1
  Demux/1 -> Terminator/1  "phi"
  Demux/2 -> Trigonometric Function1/1  "theta"
  Demux/3 -> Trigonometric Function3/1  "psi"
  Trigonometric Function1/1 -> Product/1
  Trigonometric Function3/1 -> Product/2
  Product/1 -> R_12/1

== system Sim_Multi/True dynamic system representation of a multirotor UAV/Force//Moment computation/Forces and moments generated by spinning propellers/For Each Subsystem/Thrust//moment vector for each propeller (Body axes)/Coordinate transformation Body to Motor axes/Rotation Matrix Body to Motor/Subsystem2 ==
  Euler : Inport
  Demux : Demux  Outputs=3
  Gain : Gain  Gain=-1
  Terminator : Terminator
  Terminator1 : Terminator
  Trigonometric Function1 : Trigonometry
  R_13 : Outport
  wires:
  Euler/1 -> Demux/1
  Demux/1 -> Terminator/1  "phi"
  Demux/2 -> Trigonometric Function1/1  "theta"
  Demux/3 -> Terminator1/1  "psi"
  Trigonometric Function1/1 -> Gain/1
  Gain/1 -> R_13/1

== system Sim_Multi/True dynamic system representation of a multirotor UAV/Force//Moment computation/Forces and moments generated by spinning propellers/For Each Subsystem/Thrust//moment vector for each propeller (Body axes)/Coordinate transformation Body to Motor axes/Rotation Matrix Body to Motor/Subsystem3 ==
  Euler : Inport
  Demux : Demux  Outputs=3
  Product : Product  Inputs=3
  Product1 : Product
  Sum : Sum  Inputs=|+-
  Trigonometric Function : Trigonometry
  Trigonometric Function1 : Trigonometry
  Trigonometric Function12 : Trigonometry
  Trigonometric Function3 : Trigonometry  Operator=cos
  Trigonometric Function5 : Trigonometry  Operator=cos
  R_21 : Outport
  wires:
  Euler/1 -> Demux/1
  Demux/2 -> Trigonometric Function1/1  "theta"
  Demux/3 -> Trigonometric Function/1, Trigonometric Function3/1  "psi"
  Trigonometric Function3/1 -> Product/3
  Trigonometric Function1/1 -> Product/2
  Demux/1 -> Trigonometric Function5/1, Trigonometric Function12/1  "phi"
  Trigonometric Function12/1 -> Product/1
  Trigonometric Function5/1 -> Product1/1
  Trigonometric Function/1 -> Product1/2
  Product/1 -> Sum/1
  Sum/1 -> R_21/1
  Product1/1 -> Sum/2

== system Sim_Multi/True dynamic system representation of a multirotor UAV/Force//Moment computation/Forces and moments generated by spinning propellers/For Each Subsystem/Thrust//moment vector for each propeller (Body axes)/Coordinate transformation Body to Motor axes/Rotation Matrix Body to Motor/Subsystem4 ==
  Euler : Inport
  Demux1 : Demux  Outputs=3
  Product1 : Product  Inputs=3
  Product2 : Product
  Sum : Sum  Inputs=|++
  Trigonometric Function : Trigonometry  Operator=cos
  Trigonometric Function12 : Trigonometry
  Trigonometric Function2 : Trigonometry
  Trigonometric Function4 : Trigonometry
  Trigonometric Function5 : Trigonometry  Operator=cos
  R_22 : Outport
  wires:
  Euler/1 -> Demux1/1
  Demux1/2 -> Trigonometric Function2/1  "theta"
  Demux1/3 -> Trigonometric Function/1, Trigonometric Function4/1  "psi"
  Trigonometric Function4/1 -> Product1/3
  Trigonometric Function2/1 -> Product1/2
  Demux1/1 -> Trigonometric Function5/1, Trigonometric Function12/1  "phi"
  Trigonometric Function12/1 -> Product1/1
  Trigonometric Function5/1 -> Product2/1
  Trigonometric Function/1 -> Product2/2
  Product1/1 -> Sum/1
  Sum/1 -> R_22/1
  Product2/1 -> Sum/2

== system Sim_Multi/True dynamic system representation of a multirotor UAV/Force//Moment computation/Forces and moments generated by spinning propellers/For Each Subsystem/Thrust//moment vector for each propeller (Body axes)/Coordinate transformation Body to Motor axes/Rotation Matrix Body to Motor/Subsystem5 ==
  Euler : Inport
  Demux : Demux  Outputs=3
  Product : Product
  Terminator : Terminator
  Trigonometric Function1 : Trigonometry  Operator=cos
  Trigonometric Function3 : Trigonometry
  R_23 : Outport
  wires:
  Euler/1 -> Demux/1
  Demux/2 -> Trigonometric Function1/1  "theta"
  Product/1 -> R_23/1
  Demux/1 -> Trigonometric Function3/1  "phi"
  Demux/3 -> Terminator/1  "psi"
  Trigonometric Function3/1 -> Product/1
  Trigonometric Function1/1 -> Product/2

== system Sim_Multi/True dynamic system representation of a multirotor UAV/Force//Moment computation/Forces and moments generated by spinning propellers/For Each Subsystem/Thrust//moment vector for each propeller (Body axes)/Coordinate transformation Body to Motor axes/Rotation Matrix Body to Motor/Subsystem6 ==
  Euler : Inport
  Demux1 : Demux  Outputs=3
  Product1 : Product  Inputs=3
  Product2 : Product
  Sum : Sum  Inputs=|++
  Trigonometric Function : Trigonometry
  Trigonometric Function12 : Trigonometry  Operator=cos
  Trigonometric Function2 : Trigonometry
  Trigonometric Function4 : Trigonometry  Operator=cos
  Trigonometric Function5 : Trigonometry
  R_31 : Outport
  wires:
  Euler/1 -> Demux1/1
  Demux1/2 -> Trigonometric Function2/1  "theta"
  Demux1/3 -> Trigonometric Function/1, Trigonometric Function4/1  "psi"
  Trigonometric Function4/1 -> Product1/3
  Trigonometric Function2/1 -> Product1/2
  Demux1/1 -> Trigonometric Function5/1, Trigonometric Function12/1  "phi"
  Trigonometric Function12/1 -> Product1/1
  Trigonometric Function5/1 -> Product2/1
  Trigonometric Function/1 -> Product2/2
  Product1/1 -> Sum/1
  Sum/1 -> R_31/1
  Product2/1 -> Sum/2

== system Sim_Multi/True dynamic system representation of a multirotor UAV/Force//Moment computation/Forces and moments generated by spinning propellers/For Each Subsystem/Thrust//moment vector for each propeller (Body axes)/Coordinate transformation Body to Motor axes/Rotation Matrix Body to Motor/Subsystem7 ==
  Euler : Inport
  Demux : Demux  Outputs=3
  Product : Product  Inputs=3
  Product1 : Product
  Sum : Sum  Inputs=|+-
  Trigonometric Function : Trigonometry  Operator=cos
  Trigonometric Function1 : Trigonometry
  Trigonometric Function12 : Trigonometry  Operator=cos
  Trigonometric Function3 : Trigonometry
  Trigonometric Function5 : Trigonometry
  R_32 : Outport
  wires:
  Euler/1 -> Demux/1
  Demux/2 -> Trigonometric Function1/1  "theta"
  Demux/3 -> Trigonometric Function/1, Trigonometric Function3/1  "psi"
  Trigonometric Function3/1 -> Product/3
  Trigonometric Function1/1 -> Product/2
  Demux/1 -> Trigonometric Function5/1, Trigonometric Function12/1  "phi"
  Trigonometric Function12/1 -> Product/1
  Trigonometric Function5/1 -> Product1/1
  Trigonometric Function/1 -> Product1/2
  Product/1 -> Sum/1
  Sum/1 -> R_32/1
  Product1/1 -> Sum/2

== system Sim_Multi/True dynamic system representation of a multirotor UAV/Force//Moment computation/Forces and moments generated by spinning propellers/For Each Subsystem/Thrust//moment vector for each propeller (Body axes)/Coordinate transformation Body to Motor axes/Rotation Matrix Body to Motor/Subsystem8 ==
  Euler : Inport
  Demux : Demux  Outputs=3
  Product : Product
  Terminator : Terminator
  Trigonometric Function1 : Trigonometry  Operator=cos
  Trigonometric Function3 : Trigonometry  Operator=cos
  R_33 : Outport
  wires:
  Euler/1 -> Demux/1
  Demux/2 -> Trigonometric Function1/1  "theta"
  Product/1 -> R_33/1
  Demux/3 -> Terminator/1  "psi"
  Demux/1 -> Trigonometric Function3/1  "phi"
  Trigonometric Function3/1 -> Product/1
  Trigonometric Function1/1 -> Product/2

== system Sim_Multi/True dynamic system representation of a multirotor UAV/Force//Moment computation/Forces and moments generated by spinning propellers/For Each Subsystem/Thrust//moment vector for each propeller (Body axes)/Coordinate transformation Body to Motor axes/Rotation Matrix Body to Motor/Subsystem9 ==
  R_11 : Inport  PortDimensions=1
  R_12 : Inport  Port=2  PortDimensions=1
  R_13 : Inport  Port=3  PortDimensions=1
  R_21 : Inport  Port=4  PortDimensions=1
  R_22 : Inport  Port=5  PortDimensions=1
  R_23 : Inport  Port=6  PortDimensions=1
  R_31 : Inport  Port=7  PortDimensions=1
  R_32 : Inport  Port=8  PortDimensions=1
  R_33 : Inport  Port=9  PortDimensions=1
  Reshape (9) to [3x3] column-major : Reshape  OutputDimensionality=Customize  OutputDimensions=[3,3]
  Vector Concatenate : Concatenate  NumInputs=9
  R_mb : Outport
  wires:
  R_33/1 -> Vector Concatenate/9
  R_22/1 -> Vector Concatenate/5
  Reshape (9) to [3x3] column-major/1 -> R_mb/1
  R_11/1 -> Vector Concatenate/1
  Vector Concatenate/1 -> Reshape (9) to [3x3] column-major/1
  R_32/1 -> Vector Concatenate/6
  R_31/1 -> Vector Concatenate/3
  R_21/1 -> Vector Concatenate/2
  R_13/1 -> Vector Concatenate/7
  R_12/1 -> Vector Concatenate/4
  R_23/1 -> Vector Concatenate/8

== system Sim_Multi/True dynamic system representation of a multirotor UAV/Force//Moment computation/Compute aerodynamic drag of the airframe in Body axes/Aerodynamic drag force/Nonzero airspeed/Surface area computation/Surface area computation/norm/dot_product ==
  u : Inport
  v : Inport  Port=2
  Product : Product  Multiplication=Matrix(*)  RndMeth=Zero
  Reshape : Reshape  OutputDimensionality=Column vector (2-D)
  Reshape1 : Reshape  OutputDimensionality=Column vector (2-D)
  transpose : Math  Operator=transpose  SaturateOnIntegerOverflow=on
  u.v : Outport
  wires:
  v/1 -> Reshape1/1
  u/1 -> Reshape/1
  Reshape/1 -> transpose/1
  transpose/1 -> Product/1
  Reshape1/1 -> Product/2
  Product/1 -> u.v/1

== system Sim_Multi/True dynamic system representation of a multirotor UAV/Force//Moment computation/Forces and moments generated by spinning propellers/For Each Subsystem/Thrust//moment vector for each propeller (Body axes)/Compute dynamic motor thrust and moments/Blade flapping computations/Nonzero airspeed in rotor plane/norm ==
  u : Inport
  Complex to Real-Imag : ComplexToRealImag  Output=Real
  Sqrt : Sqrt  SaturateOnIntegerOverflow=on
  dot_product : Subsystem
  ||u|| : Outport
  wires:
  u/1 -> dot_product/1(u), dot_product/2(v)
  dot_product/1(u.v) -> Sqrt/1
  Sqrt/1 -> Complex to Real-Imag/1
  Complex to Real-Imag/1 -> ||u||/1

== system Sim_Multi/True dynamic system representation of a multirotor UAV/Force//Moment computation/Forces and moments generated by spinning propellers/For Each Subsystem/Thrust//moment vector for each propeller (Body axes)/Compute dynamic motor thrust and moments/Blade flapping computations/norm/dot_product ==
  u : Inport
  v : Inport  Port=2
  Product : Product  Multiplication=Matrix(*)  RndMeth=Zero
  Reshape : Reshape  OutputDimensionality=Column vector (2-D)
  Reshape1 : Reshape  OutputDimensionality=Column vector (2-D)
  transpose : Math  Operator=transpose  SaturateOnIntegerOverflow=on
  u.v : Outport
  wires:
  v/1 -> Reshape1/1
  u/1 -> Reshape/1
  Reshape/1 -> transpose/1
  transpose/1 -> Product/1
  Reshape1/1 -> Product/2
  Product/1 -> u.v/1
